simulink model "Model_XSA"  (Simulink 3.00)
settings: Solver=ode45  StartTime="    0.0167"  StopTime=7.6  MaxStep=0.001  RelTol=1e-3  AbsTol=1e-3
values from neighbouring files (symbols this model uses):
  Ad = [Adop(1); A]    [sa_ta_optim.m]    (also in sur_opt.m)
  F = ec1807kf(ndx,6)    [sa_ta_optim.m]    (also in sur_opt.m)
  K1 = par(3)    [error_sa_ta.m]    (also in sa_ta_optim.m = par1(3); sur_opt.m = xm(3))
  Ks = par(2)    [error_sa_ta.m]    (also in sa_ta_optim.m = par1(2); sur_opt.m = xm(2))
  Mmax = par(1)    [error_sa_ta.m]    (also in sa_ta_optim.m = par1(1); sur_opt.m = xm(1))
  Sd = ec1807kf(ndx,2)    [sa_ta_optim.m]    (also in sur_opt.m = interp1(t, Sd, Tt1))
  V = ec1807k(ndx,6)    [sa_ta_optim.m]    (also in sur_opt.m)
  Xd = ec1807kf(ndx,3)    [sa_ta_optim.m]    (also in sur_opt.m = interp1(t, Xd, Tt1))
undefined symbols (not defined in the file or in its folder): K2
settings Model: SaveTime=off  SaveOutput=off  LastModifiedBy=ME

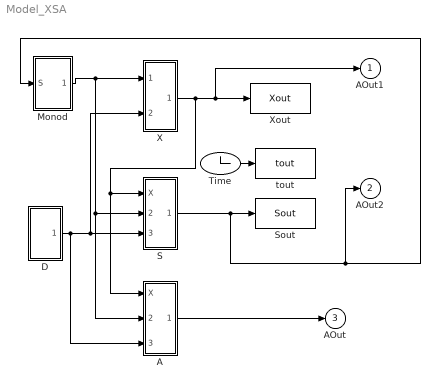
== system Model_XSA ==
  A : Subsystem
  D : Subsystem
  Monod : Subsystem
  S : Subsystem
  Sout : ToWorkspace  VariableName=Sout  SampleTime=-1  SaveFormat=Matrix
      settings: Buffer=1000
  Time : Clock
      settings: Decimation=10
  X : Subsystem
  Xout : ToWorkspace  VariableName=Xout  SampleTime=-1  SaveFormat=Matrix
      settings: Buffer=1000
  tout : ToWorkspace  VariableName=tout  SampleTime=-1  SaveFormat=Matrix
      settings: Buffer=1000
  AOut1 : Outport  Port=1
  AOut2 : Outport  Port=2
  AOut : Outport  Port=3
  wires:
  X/1(XOut) -> S/1(X), A/1(X), Xout/1, AOut1/1
  Time/1 -> tout/1
  Monod/1(mu) -> X/1(mu), S/2(mu), A/2(mu)
  D/1(out_1) -> S/3(F/V), X/2(F/V), A/3(F/V)
  S/1(Sout) -> Sout/1, AOut2/1, Monod/1(S)
  A/1(Aout) -> AOut/1

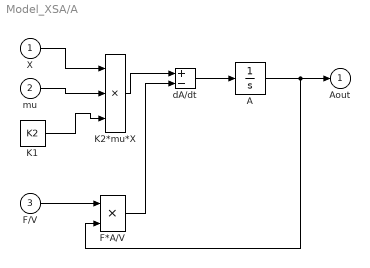
== system Model_XSA/A ==
  X : Inport  Port=1  PortWidth=-1  SampleTime=-1  DataType=auto
      settings: SignalType=auto
  mu : Inport  Port=2  PortWidth=-1  SampleTime=-1  DataType=auto
      settings: SignalType=auto
  F/V : Inport  Port=3  PortWidth=-1  SampleTime=-1  DataType=auto
      settings: SignalType=auto
  A : Integrator  ExternalReset=none  InitialConditionSource=internal  InitialCondition=Ad(1)  LimitOutput=off  UpperSaturationLimit=inf  LowerSaturationLimit=-inf  ShowSaturationPort=off  ShowStatePort=off  AbsoluteTolerance=auto
  F*A/V : Product  Inputs=2  SaturateOnIntegerOverflow=on
  K1 : Constant  Value=K2
  K2*mu*X : Product  Inputs=3  SaturateOnIntegerOverflow=on
  dA/dt : Sum  Inputs=+-  SaturateOnIntegerOverflow=on
  Aout : Outport  Port=1
  wires:
  A/1 -> Aout/1, F*A/V/2
  dA/dt/1 -> A/1
  K2*mu*X/1 -> dA/dt/1
  X/1 -> K2*mu*X/1
  mu/1 -> K2*mu*X/2
  F/V/1 -> F*A/V/1
  F*A/V/1 -> dA/dt/2
  K1/1 -> K2*mu*X/3

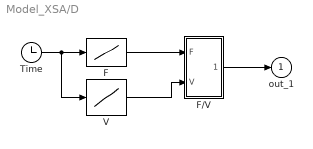
== system Model_XSA/D ==
  F : Lookup  InputValues=t  OutputValues=F
  F/V : Subsystem
      mask Type: /
      mask Description: Division of two scalars. y=u[1]/u[2]
      mask Help: Division of two scalars: y=u[1]/u[2]
      mask Display: disp('/')
  Time : Clock
      settings: DisplayTime=off  Decimation=10
  V : Lookup  InputValues=t  OutputValues=V
  out_1 : Outport  Port=1
  wires:
  F/V/1(out_1) -> out_1/1
  F/1 -> F/V/1(F)
  V/1 -> F/V/2(V)
  Time/1 -> F/1, V/1

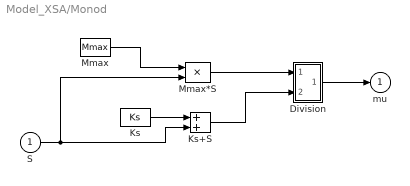
== system Model_XSA/Monod ==
  S : Inport  Port=1  PortWidth=-1  SampleTime=-1  DataType=auto
      settings: SignalType=auto
  Division : Subsystem
      mask Type: /
      mask Description: Division of two scalars. y=u[1]/u[2]
      mask Help: Division of two scalars: y=u[1]/u[2]
      mask Display: disp('/')
  Ks : Constant  Value=Ks
  Ks+S : Sum  Inputs=++  SaturateOnIntegerOverflow=on
  Mmax : Constant  Value=Mmax
  Mmax*S : Product  Inputs=2  SaturateOnIntegerOverflow=on
  mu : Outport  Port=1
  wires:
  Mmax/1 -> Mmax*S/1
  Mmax*S/1 -> Division/1(Mmax*S)
  Ks+S/1 -> Division/2(Ks+S)
  Ks/1 -> Ks+S/1
  S/1 -> Ks+S/2, Mmax*S/2
  Division/1(out_1) -> mu/1

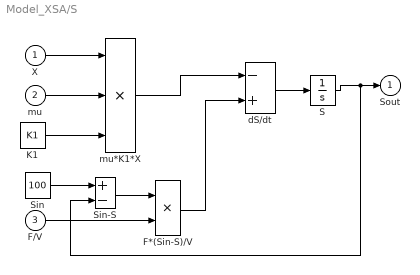
== system Model_XSA/S ==
  X : Inport  Port=1  PortWidth=-1  SampleTime=-1  DataType=auto
      settings: SignalType=auto
  mu : Inport  Port=2  PortWidth=-1  SampleTime=-1  DataType=auto
      settings: SignalType=auto
  F/V : Inport  Port=3  PortWidth=-1  SampleTime=-1  DataType=auto
      settings: SignalType=auto
  F*(Sin-S)/V : Product  Inputs=2  SaturateOnIntegerOverflow=on
  K1 : Constant  Value=K1
  S : Integrator  ExternalReset=none  InitialConditionSource=internal  InitialCondition=Sd(1)  LimitOutput=off  UpperSaturationLimit=1000  LowerSaturationLimit=0  ShowSaturationPort=off  ShowStatePort=off  AbsoluteTolerance=auto
  Sin : Constant  Value=100
  Sin-S : Sum  Inputs=+-  SaturateOnIntegerOverflow=on
  dS/dt : Sum  Inputs=-+  SaturateOnIntegerOverflow=on
  mu*K1*X : Product  Inputs=3  SaturateOnIntegerOverflow=on
  Sout : Outport  Port=1
  wires:
  S/1 -> Sout/1, Sin-S/2
  Sin-S/1 -> F*(Sin-S)/V/1
  Sin/1 -> Sin-S/1
  X/1 -> mu*K1*X/1
  F/V/1 -> F*(Sin-S)/V/2
  mu*K1*X/1 -> dS/dt/1
  F*(Sin-S)/V/1 -> dS/dt/2
  dS/dt/1 -> S/1
  mu/1 -> mu*K1*X/2
  K1/1 -> mu*K1*X/3

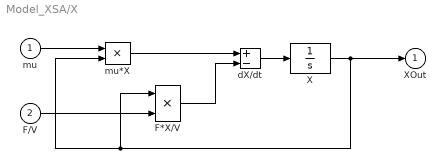
== system Model_XSA/X ==
  mu : Inport  Port=1  PortWidth=-1  SampleTime=-1  DataType=auto
      settings: SignalType=auto
  F/V : Inport  Port=2  PortWidth=-1  SampleTime=-1  DataType=auto
      settings: SignalType=auto
  F*X/V : Product  Inputs=2  SaturateOnIntegerOverflow=on
  X : Integrator  ExternalReset=none  InitialConditionSource=internal  InitialCondition=Xd(1)  LimitOutput=off  UpperSaturationLimit=1000  LowerSaturationLimit=0  ShowSaturationPort=off  ShowStatePort=off  AbsoluteTolerance=auto
  dX/dt : Sum  Inputs=+-  SaturateOnIntegerOverflow=on
  mu*X : Product  Inputs=2  SaturateOnIntegerOverflow=on
  XOut : Outport  Port=1
  wires:
  F*X/V/1 -> dX/dt/2
  dX/dt/1 -> X/1
  mu*X/1 -> dX/dt/1
  mu/1 -> mu*X/1
  X/1 -> XOut/1, mu*X/2, F*X/V/1
  F/V/1 -> F*X/V/2

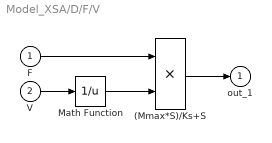
== system Model_XSA/D/F/V ==
  F : Inport  Port=1  PortWidth=-1  SampleTime=-1  DataType=auto
      settings: SignalType=auto
  V : Inport  Port=2  PortWidth=-1  SampleTime=-1  DataType=auto
      settings: SignalType=auto
  (Mmax*S)/Ks+S : Product  Inputs=2  SaturateOnIntegerOverflow=on
  Math Function : Math  Operator=reciprocal  OutputSignalType=auto
  out_1 : Outport  Port=1
  wires:
  F/1 -> (Mmax*S)/Ks+S/1
  V/1 -> Math Function/1
  Math Function/1 -> (Mmax*S)/Ks+S/2
  (Mmax*S)/Ks+S/1 -> out_1/1

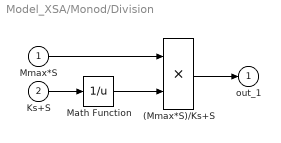
== system Model_XSA/Monod/Division ==
  Mmax*S : Inport  Port=1  PortWidth=-1  SampleTime=-1  DataType=auto
      settings: SignalType=auto
  Ks+S : Inport  Port=2  PortWidth=-1  SampleTime=-1  DataType=auto
      settings: SignalType=auto
  (Mmax*S)/Ks+S : Product  Inputs=2  SaturateOnIntegerOverflow=on
  Math Function : Math  Operator=reciprocal  OutputSignalType=auto
  out_1 : Outport  Port=1
  wires:
  Mmax*S/1 -> (Mmax*S)/Ks+S/1
  Ks+S/1 -> Math Function/1
  Math Function/1 -> (Mmax*S)/Ks+S/2
  (Mmax*S)/Ks+S/1 -> out_1/1
